simulink model "fixpt_numerictype"  (R2015b)
settings: Solver=ode45  StartTime=0.0  StopTime=10.0  RelTol=1e-3
PreLoadFcn:
  | mydt = fixdt(1,8,4)
settings Model: Creator=at-mt  LastModifiedBy=amatsumo
settings DataIOCC: SaveFormat=Array  SignalLoggingSaveFormat=ModelDataLogs
settings OptimizationCC: ExpressionDepthLimit=2147483647  InitFltsAndDblsToZero=on
settings DebuggingCC: UnderspecifiedInitializationDetection=Classic  MergeDetectMultiDrivingBlocksExec=none  SolverPrmCheckMsg=warning  FcnCallInpInsideContextMsg=UseLocalSettings  StateNameClashWarn=warning
settings HardwareCC: ProdBitPerPointer=32  ProdLargestAtomicFloat=None  ProdIntDivRoundTo=Undefined  ProdEndianess=Unspecified  ProdWordSize=32  ProdHWDeviceType=32-bit Generic
settings GRTTargetCC: GeneratePreprocessorConditionals=Disable all  CombineOutputUpdateFcns=off  GRTInterface=on
settings ConfigComp: CovModelRefEnable=Off  CovSFcnEnable=off

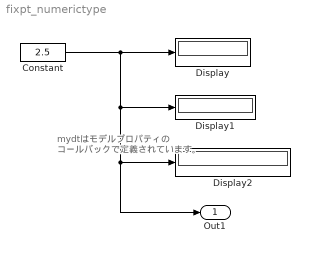
== system fixpt_numerictype ==
  note: mydtはモデルプロパティの
      | コールバックで定義されています。
  Constant : Constant  Value=2.5  OutDataTypeStr=mydt  SampleTime=-1
      settings: AttributesFormatString=DataType = %<OutDataTypeStr>
  Display : Display
      settings: AttributesFormatString=Format = %<Format>
  Display1 : Display
      settings: AttributesFormatString=Format = %<Format>  Format=hex (Stored Integer)
  Display2 : Display
      settings: AttributesFormatString=Format = %<Format>  Format=binary (Stored Integer)
  Out1 : Outport
  wires:
  Constant/1 -> Display2/1, Out1/1, Display1/1, Display/1
